simulink model "my_spwm_controller"  (R2020a)
settings: Solver=ode23tb  StartTime=0.0  StopTime=0.1  MaxStep=0.00001  RelTol=1e-3  EnableMultiTasking=on
InitFcn:
  | f=50;
  | Mf=100;
  | Fc=f*Mf;
  | Vdc=500;
  | T_dead=11e-6;
libraries: dsparch4 x3, simulink x1, powerlib x1
settings Model: Creator=Lei  LastModifiedBy=DELL
settings DataIOCC: LimitDataPoints=on  SaveFormat=Array  ReturnWorkspaceOutputs=off
settings OptimizationCC: LifeSpan=inf
settings DebuggingCC: SolverPrmCheckMsg=warning  SFUnexpectedBacktrackingDiag=warning  SFNoUnconditionalDefaultTransitionDiag=warning  ArithmeticOperatorsInVariantConditions=warning
settings HardwareCC: ProdBitPerPointer=32  ProdBitPerSizeT=32  ProdBitPerPtrDiffT=32  ProdLargestAtomicFloat=None  ProdIntDivRoundTo=Undefined  ProdEndianess=Unspecified  ProdWordSize=32  ProdHWDeviceType=32-bit Generic
settings ModelReferenceCC: PropagateSignalLabelsOutOfModel=off
settings SFSimCC: SimUseLocalCustomCode=off  CustomCodeUndefinedFunction=UseInterfaceOnly
settings RTWCC: RTWUseLocalCustomCode=off
settings CodeAppCC: StateflowObjectComments=on
settings GRTTargetCC: TargetLangStandard=C89/C90 (ANSI)
settings ConfigComp: CovMetricSettings=dw  CovHtmlReporting=on  CovSaveCumulativeToWorkspaceVar=on  CovSaveSingleToWorkspaceVar=on  CovExternalEMLEnable=off  CovSFcnEnable=off
settings SimscapeCC: SimscapeNormalizeSystem=off
settings ConfigurationSet: Description=SimMechanics 2G

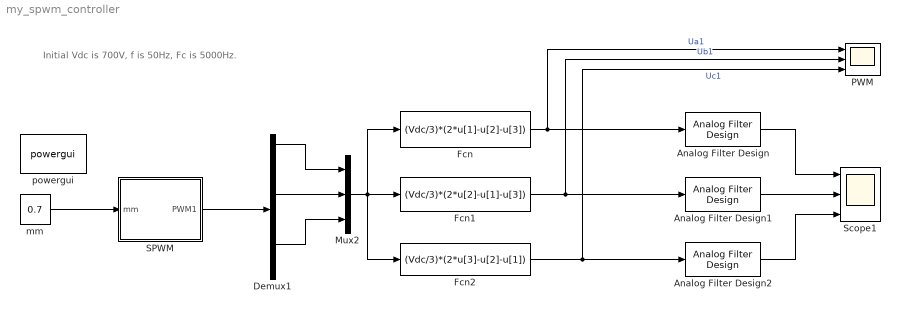
== system my_spwm_controller ==
  note: Initial Vdc is 700V, f is 50Hz, Fc is 5000Hz.
  Analog Filter Design : dsparch4/Analog Filter Design  method=Butterworth  filttype=Lowpass  N=4  Wlo=5*2*pi*f  Whi=80  Rp=2  Rs=40
  Analog Filter Design1 : dsparch4/Analog Filter Design  method=Butterworth  filttype=Lowpass  N=4  Wlo=5*2*pi*f  Whi=80  Rp=2  Rs=40
  Analog Filter Design2 : dsparch4/Analog Filter Design  method=Butterworth  filttype=Lowpass  N=4  Wlo=5*2*pi*f  Whi=80  Rp=2  Rs=40
  Demux1 : Demux  Outputs=6
  Fcn : Fcn  Expr=(Vdc/3)*(2*u[1]-u[2]-u[3])
  Fcn1 : Fcn  Expr=(Vdc/3)*(2*u[2]-u[1]-u[3])
  Fcn2 : Fcn  Expr=(Vdc/3)*(2*u[3]-u[2]-u[1])
  Mux2 : Mux  Inputs=3
  PWM : Scope  NumInputPorts=3
  SPWM : Subsystem
  Scope1 : Scope  NumInputPorts=3
  mm : Constant  Value=0.7
  powergui : powerlib/powergui  Priority=1  SimulationMode=Discrete  SampleTime=50e-6  frequency=60  Iterations=50  frequencyindice=60  Pbase=100e6  ErrMax=1e-4  UnitsV=kV  UnitsW=MW  buscounter=0  FunctionMessages=off  echomessages=off  EnableUseOfTLC=off  CurrentSourceSwitches=on  DisableSnubberDevices=off  DisableRonSwitches=off  DisableVfSwitches=off  DisplayEquations=off  AutomaticDiscreteSolvers=off  SolverType=Tustin/Backward Euler (TBE)  Interpol=off  ExternalGateDelay=off  methode=off  Ts=100  x0status=blocks  SPID=off  SwTol=0  HookPort=off  NonlinearTolerance=1e-4  nMaxIteration=100  ContinueOnMaxIteration=off  RestoreLinks=warning  ResistiveCurrentMeasurement=off  Frange=[0:2:500]  Ylog=off  Xlog=on  ShowGrid=off  save=off  variable=ZData  structure=Ua_  ZoomFFT=off  StartTime=0.07  cycles=1  DisplayStyle=1  fundamental=50  FreqAxis=off  MaxFrequency=9000  frequencyindicesteady=1  RmsSteady=1  display=off
  wires:
  Mux2/1 -> Fcn/1, Fcn2/1, Fcn1/1
  Demux1/3 -> Mux2/2
  Demux1/5 -> Mux2/3
  Demux1/1 -> Mux2/1
  Fcn1/1 -> Analog Filter Design1/1, PWM/2  "Ub1"
  Fcn/1 -> Analog Filter Design/1, PWM/1  "Ua1"
  Fcn2/1 -> Analog Filter Design2/1, PWM/3  "Uc1"
  mm/1 -> SPWM/1(mm)
  SPWM/1(PWM1) -> Demux1/1
  Analog Filter Design1/1 -> Scope1/2
  Analog Filter Design2/1 -> Scope1/3
  Analog Filter Design/1 -> Scope1/1

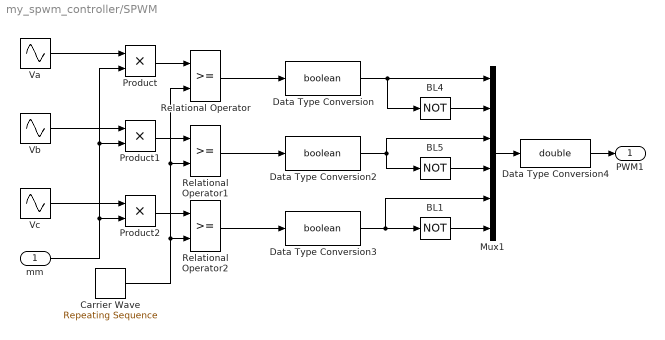
== system my_spwm_controller/SPWM ==
  mm : Inport
  BL1 : Logic  Operator=NOT  Inputs=1
  BL4 : Logic  Operator=NOT  Inputs=1
  BL5 : Logic  Operator=NOT  Inputs=1
  Carrier Wave : simulink/Sources/Repeating Sequence  rep_seq_t=[0 1/Fc/4 3/Fc/4 1/Fc]  rep_seq_y=[0 -1 1 0]
  Data Type Conversion4 : DataTypeConversion  OutDataTypeStr=double  SaturateOnIntegerOverflow=on  RndMeth=Zero
  Data Type Conversion : DataTypeConversion  OutDataTypeStr=boolean  SaturateOnIntegerOverflow=on  RndMeth=Zero
  Data Type Conversion2 : DataTypeConversion  OutDataTypeStr=boolean  SaturateOnIntegerOverflow=on  RndMeth=Zero
  Data Type Conversion3 : DataTypeConversion  OutDataTypeStr=boolean  SaturateOnIntegerOverflow=on  RndMeth=Zero
  Mux1 : Mux  Inputs=6
  Product : Product
  Product1 : Product
  Product2 : Product
  Relational Operator : RelationalOperator  RndMeth=Nearest  InputSameDT=on
  Relational Operator1 : RelationalOperator  RndMeth=Nearest  InputSameDT=on
  Relational Operator2 : RelationalOperator  RndMeth=Nearest  InputSameDT=on
  Va : Sin  Frequency=2*pi*f  SampleTime=0
  Vb : Sin  Frequency=2*pi*f  Phase=-2*pi/3  SampleTime=0
  Vc : Sin  Frequency=2*pi*f  Phase=-4*pi/3  SampleTime=0
  PWM1 : Outport
  wires:
  Vc/1 -> Product2/1
  Va/1 -> Product/1
  Product/1 -> Relational Operator/1
  mm/1 -> Product2/2, Product1/2, Product/2
  Data Type Conversion2/1 -> Mux1/3, BL5/1
  Vb/1 -> Product1/1
  Product1/1 -> Relational Operator1/1
  Carrier Wave/1 -> Relational Operator1/2, Relational Operator/2, Relational Operator2/2
  Data Type Conversion/1 -> Mux1/1, BL4/1
  BL4/1 -> Mux1/2
  Product2/1 -> Relational Operator2/1
  BL1/1 -> Mux1/6
  BL5/1 -> Mux1/4
  Data Type Conversion3/1 -> Mux1/5, BL1/1
  Mux1/1 -> Data Type Conversion4/1
  Relational Operator/1 -> Data Type Conversion/1
  Data Type Conversion4/1 -> PWM1/1
  Relational Operator1/1 -> Data Type Conversion2/1
  Relational Operator2/1 -> Data Type Conversion3/1
